simulink model "sis_sus"  (R2019a)
settings: Solver=VariableStepAuto  StartTime=0.0  StopTime=30  RelTol=1e-3
values from neighbouring files (symbols this model uses):
  b = 10    [sis_mec.m]    (also in sis_sus_vehiculo.m = 500)
  k1 = 300    [sis_sus_vehiculo.m]
  k2 = 50    [sis_sus_vehiculo.m]
  m1 = 10    [sis_sus_vehiculo.m]
  m2 = 400    [sis_sus_vehiculo.m]
settings Model: Creator=cmparedes  LastModifiedBy=cmparedes

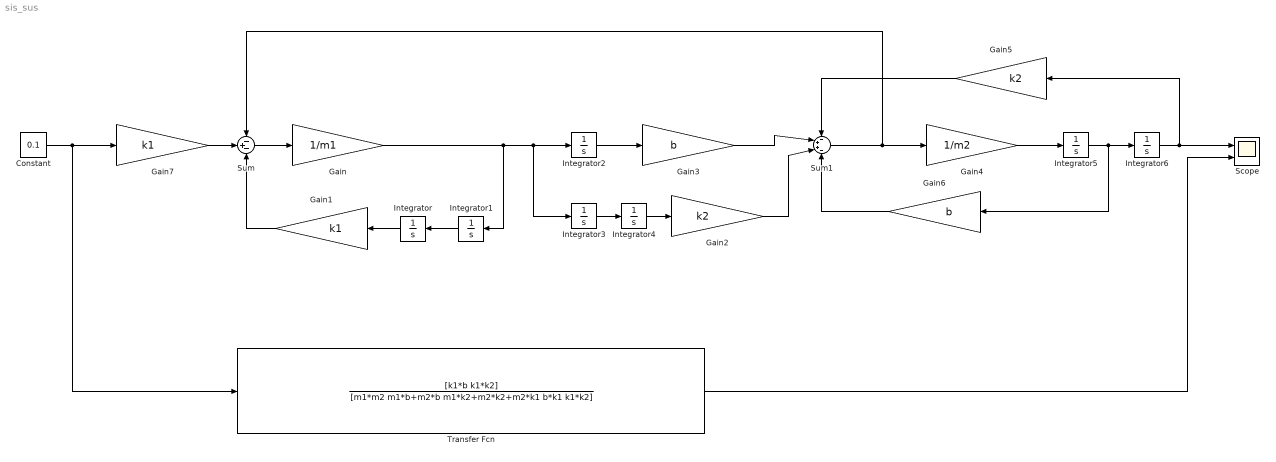
== system sis_sus ==
  Constant : Constant  Value=0.1
  Gain : Gain  Gain=1/m1
  Gain1 : Gain  Gain=k1
  Gain2 : Gain  Gain=k2
  Gain3 : Gain  Gain=b
  Gain4 : Gain  Gain=1/m2
  Gain5 : Gain  Gain=k2
  Gain6 : Gain  Gain=b
  Gain7 : Gain  Gain=k1
  Integrator{,1..6} (7 alike) : Integrator
  Scope : Scope  NumInputPorts=2
  Sum : Sum  Inputs=-+-
  Sum1 : Sum  Inputs=-++-
  Transfer Fcn : TransferFcn  Numerator=[k1*b k1*k2]  Denominator=[m1*m2 m1*b+m2*b m1*k2+m2*k2+m2*k1 b*k1 k1*k2]
  wires:
  Sum/1 -> Gain/1
  Integrator/1 -> Gain1/1
  Integrator1/1 -> Integrator/1
  Gain/1 -> Integrator3/1, Integrator2/1, Integrator1/1
  Integrator3/1 -> Integrator4/1
  Integrator4/1 -> Gain2/1
  Integrator2/1 -> Gain3/1
  Gain1/1 -> Sum/3
  Gain2/1 -> Sum1/3
  Gain3/1 -> Sum1/2
  Gain5/1 -> Sum1/1
  Gain6/1 -> Sum1/4
  Sum1/1 -> Gain4/1, Sum/1
  Gain4/1 -> Integrator5/1
  Integrator5/1 -> Gain6/1, Integrator6/1
  Integrator6/1 -> Gain5/1, Scope/1
  Gain7/1 -> Sum/2
  Constant/1 -> Transfer Fcn/1, Gain7/1
  Transfer Fcn/1 -> Scope/2
